simulink model "state_3_machine"  (R2017b)
settings: Solver=VariableStepAuto  StartTime=0.0  StopTime=10.0  RelTol=1e-3
settings Model: Creator=Kalana  LastModifiedBy=Kalana

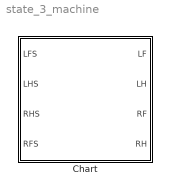
== system state_3_machine ==
  Chart : Stateflow chart  TreatAsAtomicUnit=on

== stateflow chart state_3_machine/Chart ==
  state Intermediate1
    entry: LF = 2
    RF = 1
    RH = 0
    LH = 1
  state Intermediate
    entry: LF = 0
    RF = 1
    RH = 2
    LH = 1
  state LF_RH_swing
    entry: LF = 0
    RF = 1
    RH = 0
    LH = 1
  state RF_LH_swing
    entry: LF = 1
    RF = 0
    RH = 1
    LH = 0
  state Intermediate3
    entry: LF = 1
    RF = 0
    RH = 1
    LH = 2
  state Intermediate2
    entry: LF = 1
    RF = 2
    RH = 1
    LH = 0
  LF_RH_swing -> Intermediate1 [order 1] : [LFS ]
  Intermediate1 -> RF_LH_swing : [RHS]
  Intermediate -> RF_LH_swing : [LFS]
  LF_RH_swing -> Intermediate [order 2] : [RHS]
  (default) -> LF_RH_swing
  Intermediate3 -> LF_RH_swing : [RFS]
  RF_LH_swing -> Intermediate3 [order 2] : [LHS]
  Intermediate2 -> LF_RH_swing : [LHS]
  RF_LH_swing -> Intermediate2 [order 1] : [RFS]
  data: LF output; LH output; RF output; RH output; LFS input; LHS input; RHS input; RFS input
